simulink library "Lib_Piccolo"  (R2018b)
settings: Solver=VariableStepAuto  StartTime=0.0  StopTime=10.0  RelTol=1e-3
values from neighbouring files (symbols this model uses):
  AccelErrInt2Brakes = 0.15    [SimulationControlConfig16P.m]    (also in SimulationControlConfig16P_F0.m; SimulationControlConfig16P_F2.m; SimulationControlConfig16P_LEGACY.m; SimulationControlConfigTAILLESS.m = 0.2)
  AileronMax = 25    [SimulationControlConfig16P.m]    (also in SimulationControlConfig16P_F0.m; SimulationControlConfig16P_F2.m; SimulationControlConfig16P_LEGACY.m; SimulationControlConfigTAILLESS.m)
  AileronPower = 0.00268    [SimulationControlConfig16P.m]    (also in SimulationControlConfig16P_F0.m; SimulationControlConfig16P_F2.m; SimulationControlConfig16P_LEGACY.m; SimulationControlConfigTAILLESS.m = 0.002266)
  AileronSurfaceMax = 45    [SimulationControlConfig16P.m]    (also in SimulationControlConfig16P_F0.m; SimulationControlConfig16P_F2.m; SimulationControlConfig16P_LEGACY.m; SimulationControlConfigTAILLESS_CGAFT_F0.m = 25)
  AileronTrim = 0    [SimulationControlConfig16P.m]    (also in SimulationControlConfig16P_F0.m; SimulationControlConfig16P_F2.m; SimulationControlConfig16P_LEGACY.m; SimulationControlConfigTAILLESS.m)
  Alt = 1000 + TerrainHeight    [SimulationStateConfig.m]
  AltCruise_m = Alt * 0.3048    [SimulationControlConfig16P.m]    (also in SimulationControlConfig16P_F2.m; SimulationControlConfigTAILLESS.m = Alt/3.28084; SimulationControlConfigTAILLESS_CGAFT_F0.m = 640; SimulationControlConfigTAILLESS_CGFWD_F0.m = 640)
  AltitudeRate2PitchCmdIntegratorInit = 0.1    [SimulationControlPre.m]
  AltMax = 10000    [SimulationControlConfig16P.m]    (also in SimulationControlConfig16P_F0.m; SimulationControlConfig16P_F2.m; SimulationControlConfig16P_LEGACY.m; SimulationControlConfigTAILLESS.m)
  AltMaxAccel = 2.5    [SimulationControlConfig16P.m]    (also in SimulationControlConfig16P_F0.m = 2; SimulationControlConfig16P_F2.m = 2; SimulationControlConfig16P_LEGACY.m = 0.9; SimulationControlConfigTAILLESS.m = 2)
  AltMin = 0    [SimulationControlConfig16P.m]    (also in SimulationControlConfig16P_F0.m; SimulationControlConfig16P_F2.m; SimulationControlConfig16P_LEGACY.m; SimulationControlConfigTAILLESS.m)
  AltRateCmd2Pitch = 0.26    [SimulationControlConfig16P.m]    (also in SimulationControlConfig16P_F0.m = 0.35; SimulationControlConfig16P_F2.m = 0.35; SimulationControlConfig16P_LEGACY.m = 0.6; SimulationControlConfigTAILLESS.m = 0.9)
  AltRateError2Pitch = 0.34    [SimulationControlConfig16P.m]    (also in SimulationControlConfig16P_F0.m = 0.61; SimulationControlConfig16P_F2.m = 0.61; SimulationControlConfig16P_LEGACY.m = 0.4; SimulationControlConfigTAILLESS.m = 0.3)
  AltRateErrorInt2Pitch = 0.61    [SimulationControlConfig16P.m]    (also in SimulationControlConfig16P_F0.m = 0.28; SimulationControlConfig16P_F2.m = 0.28; SimulationControlConfig16P_LEGACY.m = 0.45; SimulationControlConfigTAILLESS.m = 0.15)
  AltRateLpfCutOff = 3    [SimulationControlConfig16P.m]    (also in SimulationControlConfig16P_F0.m; SimulationControlConfig16P_F2.m; SimulationControlConfig16P_LEGACY.m; SimulationControlConfigTAILLESS.m = 5)
  AutoNosegear2Rudder = 26    [SimulationControlConfig16P.m]    (also in SimulationControlConfig16P_F0.m; SimulationControlConfig16P_F2.m; SimulationControlConfig16P_LEGACY.m; SimulationControlConfigTAILLESS.m = 25.2)
  b = 5.54    [SimulationControlConfig16P.m]    (also in SimulationControlConfig16P_F0.m; SimulationControlConfig16P_F2.m; SimulationControlConfig16P_LEGACY.m; SimulationControlConfigTAILLESS.m = 2.37)
  Bank2AileronIntegratorInit = 0    [SimulationControlPre.m]
  BankMax_User = BankMax_User/180*pi    (= 0.610865238198)    [SimulationControlConfig16P.m]    (also in SimulationControlConfig16P_F0.m = 0.523598775598; SimulationControlConfig16P_F2.m = 0.523598775598; SimulationControlConfig16P_LEGACY.m = 0.523598775598; SimulationControlConfigTAILLESS.m = 0.558505360638)
  baseLegFlaps = 20    [SimulationControlConfig16P.m]    (also in SimulationControlConfig16P_F0.m; SimulationControlConfig16P_F2.m = 15; SimulationControlConfig16P_LEGACY.m = 0; SimulationControlConfigTAILLESS.m = 0)
  C = GeneticOpt.C    [SimulationCostFunction.m]
  c = Sw/b    (= 0.841696750903)    [SimulationControlConfig16P.m]    (also in SimulationControlConfig16P_F0.m; SimulationControlConfig16P_F2.m; SimulationControlConfig16P_LEGACY.m; SimulationControlConfigTAILLESS.m = 0.354008438819)
  cell2WheelFactorMG = 5.98    [SimulationSensorConfig16P_LEGACY.m]
  cell2WheelFactorNG = 1    [SimulationSensorConfig16P_LEGACY.m]
  cellSatMaxMG = 15000    [SimulationSensorConfig16P.m]    (also in SimulationSensorConfig16P_LEGACY.m; SimulationSensorConfigTAILLESS7P.m; SimulationSensorConfigUTAIL7P.m)
  cellSatMaxNG = 1000    [SimulationSensorConfig16P.m]    (also in SimulationSensorConfig16P_LEGACY.m; SimulationSensorConfigTAILLESS7P.m; SimulationSensorConfigUTAIL7P.m)
  cellSatMinMG = -15000    [SimulationSensorConfig16P.m]    (also in SimulationSensorConfig16P_LEGACY.m; SimulationSensorConfigTAILLESS7P.m; SimulationSensorConfigUTAIL7P.m)
  cellSatMinNG = -1000    [SimulationSensorConfig16P.m]    (also in SimulationSensorConfig16P_LEGACY.m; SimulationSensorConfigTAILLESS7P.m; SimulationSensorConfigUTAIL7P.m)
  CL_Limit = CL_Max    (= 0.54)    [SimulationControlConfig16P.m]    (also in SimulationControlConfig16P_F0.m; SimulationControlConfig16P_F2.m = 0.638; SimulationControlConfig16P_LEGACY.m; SimulationControlConfigTAILLESS.m = 0.525)
  CL_Max = 0.54    [SimulationControlConfig16P.m]    (also in SimulationControlConfig16P_F0.m; SimulationControlConfig16P_F2.m = 0.638; SimulationControlConfig16P_LEGACY.m; SimulationControlConfigTAILLESS.m = 0.525)
  CL_Max_Nom = 0.465    [SimulationControlConfig16P.m]    (also in SimulationControlConfig16P_F0.m; SimulationControlConfig16P_F2.m = 0.563; SimulationControlConfig16P_LEGACY.m; SimulationControlConfigTAILLESS.m = 0.39)
  CL_Min = 0    [SimulationControlConfig16P.m]    (also in SimulationControlConfig16P_F0.m; SimulationControlConfig16P_F2.m; SimulationControlConfig16P_LEGACY.m; SimulationControlConfigTAILLESS.m)
  ClimbMaxFraction = 0.35    [SimulationControlConfig16P.m]    (also in SimulationControlConfig16P_F0.m = 0.17; SimulationControlConfig16P_F2.m = 0.17; SimulationControlConfig16P_LEGACY.m = 0.24; SimulationControlConfigTAILLESS.m = 0.21)
  ClimboutMaxBank = 7.0    (= 7)    [SimulationControlConfig16P.m]    (also in SimulationControlConfig16P_F0.m; SimulationControlConfig16P_F2.m; SimulationControlConfig16P_LEGACY.m; SimulationControlConfigTAILLESS.m = 5)
  ClimboutTimer = 7.0    (= 7)    [SimulationControlConfig16P.m]    (also in SimulationControlConfig16P_F0.m; SimulationControlConfig16P_F2.m; SimulationControlConfig16P_LEGACY.m; SimulationControlConfigTAILLESS.m)
  dCl_per_dFlap = 0.005581818    [SimulationControlConfig16P.m]    (also in SimulationControlConfig16P_F0.m = 0; SimulationControlConfig16P_F2.m = 0.0065; SimulationControlConfig16P_LEGACY.m = 0; SimulationControlConfigTAILLESS.m = 0)
  DecelerationCmd = 3.1    [SimulationControlConfig16P.m]    (also in SimulationControlConfig16P_F0.m; SimulationControlConfig16P_F2.m; SimulationControlConfig16P_LEGACY.m; SimulationControlConfigTAILLESS.m = 0.1)
  DeRotateLogicEndTimer = abs((NoseDownLimit_Deg-1)/DeRotateRamp_Dps)    [SimulationControlConfig16P.m]    (also in SimulationControlConfig16P_F0.m; SimulationControlConfig16P_F2.m; SimulationControlConfig16P_LEGACY.m; SimulationControlConfigTAILLESS.m)
  DeRotateLogicHoldNoseUpTimer = 0.1    [SimulationControlConfig16P.m]    (also in SimulationControlConfig16P_F0.m; SimulationControlConfig16P_F2.m; SimulationControlConfig16P_LEGACY.m; SimulationControlConfigTAILLESS.m)
  DeRotateLogicTimerTimeout = 2    [SimulationControlConfig16P.m]    (also in SimulationControlConfig16P_F0.m; SimulationControlConfig16P_F2.m; SimulationControlConfig16P_LEGACY.m; SimulationControlConfigTAILLESS.m)
  DeRotateLowerCmdSaturation = 0    [SimulationControlConfig16P.m]    (also in SimulationControlConfig16P_F0.m; SimulationControlConfig16P_F2.m; SimulationControlConfig16P_LEGACY.m; SimulationControlConfigTAILLESS.m)
  DeRotateRamp_Dps = 3    [SimulationControlConfig16P.m]    (also in SimulationControlConfig16P_F0.m; SimulationControlConfig16P_F2.m; SimulationControlConfig16P_LEGACY.m; SimulationControlConfigTAILLESS.m = 8)
  DeRotateUpperCmdSaturation = 7    [SimulationControlConfig16P.m]    (also in SimulationControlConfig16P_F0.m; SimulationControlConfig16P_F2.m; SimulationControlConfig16P_LEGACY.m; SimulationControlConfigTAILLESS.m)
  DescentMaxFraction = 0.22    [SimulationControlConfig16P.m]    (also in SimulationControlConfig16P_F0.m = 0.2; SimulationControlConfig16P_F2.m = 0.2; SimulationControlConfig16P_LEGACY.m = 0.2; SimulationControlConfigTAILLESS.m = 0.17)
  DesktopSimTerrainOffset_m = 0.406    [SimulationAircraftConfig.m]
  downwindFlaps = 0    [SimulationControlConfig16P.m]    (also in SimulationControlConfig16P_F0.m; SimulationControlConfig16P_F2.m = 15; SimulationControlConfig16P_LEGACY.m; SimulationControlConfigTAILLESS.m)
  downwindSplitAil = 0    [SimulationControlConfig16P_F2.m]
  DP_init = 0.5*1.225*V_init^2    [SimulationControlConfig16P.m]    (also in SimulationControlConfig16P_F0.m; SimulationControlConfig16P_F2.m; SimulationControlConfig16P_LEGACY.m; SimulationControlConfigTAILLESS.m)
  dscNoiseMG = 1    [SimulationSensorConfig16P_LEGACY.m]
  dscNoiseNG = 0.25    [SimulationSensorConfig16P_LEGACY.m]
  DSCnumBits = 24    [SimulationSensorConfig16P.m]    (also in SimulationSensorConfig16P_LEGACY.m; SimulationSensorConfigTAILLESS7P.m; SimulationSensorConfigUTAIL7P.m)
  DSCRangeMaxMG = 15000    [SimulationSensorConfig16P.m]    (also in SimulationSensorConfig16P_LEGACY.m; SimulationSensorConfigTAILLESS7P.m; SimulationSensorConfigUTAIL7P.m)
  DSCRangeMaxNG = 1000    [SimulationSensorConfig16P.m]    (also in SimulationSensorConfig16P_LEGACY.m; SimulationSensorConfigTAILLESS7P.m; SimulationSensorConfigUTAIL7P.m)
  DSCRangeMinMG = -15000    [SimulationSensorConfig16P.m]    (also in SimulationSensorConfig16P_LEGACY.m; SimulationSensorConfigTAILLESS7P.m; SimulationSensorConfigUTAIL7P.m)
  DSCRangeMinNG = -1000    [SimulationSensorConfig16P.m]    (also in SimulationSensorConfig16P_LEGACY.m; SimulationSensorConfigTAILLESS7P.m; SimulationSensorConfigUTAIL7P.m)
  dt = DLLSim.dt    [SimulationTimeStep.m]    (also in SimulationTrim.m = 0.02)
  EarlyTouchdownThreshold = 3.0    (= 3)    [SimulationControlConfig16P.m]    (also in SimulationControlConfig16P_F0.m; SimulationControlConfig16P_F2.m; SimulationControlConfig16P_LEGACY.m; SimulationControlConfigTAILLESS.m)
  ElevatorDeflectionRate = 15    [SimulationControlConfig16P.m]    (also in SimulationControlConfig16P_F0.m; SimulationControlConfig16P_F2.m; SimulationControlConfig16P_LEGACY.m = 12; SimulationControlConfigTAILLESS.m = 5)
  ElevatorMax = 25    [SimulationControlConfig16P.m]    (also in SimulationControlConfig16P_F0.m; SimulationControlConfig16P_F2.m; SimulationControlConfig16P_LEGACY.m; SimulationControlConfigTAILLESS.m)
  ElevatorPower = -0.002209    [SimulationControlConfig16P.m]    (also in SimulationControlConfig16P_F0.m; SimulationControlConfig16P_F2.m; SimulationControlConfig16P_LEGACY.m; SimulationControlConfigTAILLESS.m = -0.002668)
  ElevatorTrim = -3.5    [SimulationControlConfig16P.m]    (also in SimulationControlConfig16P_F0.m; SimulationControlConfig16P_F2.m; SimulationControlConfig16P_LEGACY.m; SimulationControlConfigTAILLESS.m = -3)
  elevonBias = 0    [SimulationControlConfig16P.m]    (also in SimulationControlConfig16P_F0.m; SimulationControlConfig16P_F2.m; SimulationControlConfig16P_LEGACY.m; SimulationControlConfigTAILLESS.m)
  Enable_TAS_Protection = 0    [SimulationControlConfig16P.m]    (also in SimulationControlConfig16P_F0.m; SimulationControlConfig16P_F2.m; SimulationControlConfig16P_LEGACY.m; SimulationControlConfigTAILLESS.m)
  EnableCrossTrackAbort = 1    [SimulationControlConfig16P.m]    (also in SimulationControlConfigTAILLESS.m; SimulationControlConfigTAILLESS_CGAFT_F0.m; SimulationControlConfigTAILLESS_CGFWD_F0.m; SimulationControlConfigTAILLESS_CGFWD_F2.m)
  EnergyBandwidth = 0.04    [SimulationControlConfig16P.m]    (also in SimulationControlConfig16P_F0.m = 0.03; SimulationControlConfig16P_F2.m = 0.03; SimulationControlConfig16P_LEGACY.m = 0.02; SimulationControlConfigTAILLESS.m = 0.06)
  EngineLhFuelCut = 0    [SimulationAircraftConfig.m]
  EngineRhFuelCut = 0    [SimulationAircraftConfig.m]
  FastThrottleRate = 0.075    [SimulationControlConfig16P.m]    (also in SimulationControlConfig16P_F0.m = 0.05; SimulationControlConfig16P_F2.m = 0.05; SimulationControlConfig16P_LEGACY.m = 0.05; SimulationControlConfigTAILLESS.m = 0.1)
  FilterWarmUpTime = 2    [SimulationSensorConfig16P.m]    (also in SimulationSensorConfig16P_LEGACY.m; SimulationSensorConfigTAILLESS7P.m; SimulationSensorConfigUTAIL7P.m)
  finalApproachFlaps = 20    [SimulationControlConfig16P.m]    (also in SimulationControlConfig16P_F0.m; SimulationControlConfig16P_F2.m = 15; SimulationControlConfig16P_LEGACY.m = 0; SimulationControlConfigTAILLESS.m = 0)
  finalApproachSplitAil = 20    [SimulationControlConfig16P_F2.m]
  FinalDescentSlope_Deg = testPlans(testIndx).descentSlope    [SimulationControlConfig16P.m]    (also in SimulationControlConfig16P_F0.m; SimulationControlConfig16P_F2.m; SimulationControlConfig16P_LEGACY.m; SimulationControlConfigTAILLESS.m)
  flapMax = 0    [SimulationControlConfig16P.m]    (also in SimulationControlConfig16P_F0.m = 35; SimulationControlConfig16P_F2.m = 33; SimulationControlConfig16P_LEGACY.m; SimulationControlConfigTAILLESS.m)
  flapRate = 7.5    [SimulationControlConfig16P.m]    (also in SimulationControlConfig16P_F0.m; SimulationControlConfig16P_F2.m; SimulationControlConfig16P_LEGACY.m; SimulationControlConfigTAILLESS.m = 6.6)
  FlareHeight = 5    [SimulationControlConfig16P.m]    (also in SimulationControlConfig16P_F0.m; SimulationControlConfig16P_F2.m; SimulationControlConfig16P_LEGACY.m = 4.8; SimulationControlConfigTAILLESS.m = 2.75)
  FlareVerticalRate_mps = -0.4    [SimulationControlConfig16P.m]    (also in SimulationControlConfig16P_F0.m; SimulationControlConfig16P_F2.m; SimulationControlConfig16P_LEGACY.m = -0.5; SimulationControlConfigTAILLESS.m = -0.15)
  Fp_Aileron = 0.55*2*pi*RollRateLpfCutoff*dt    [SimulationControlConfig16P.m]    (also in SimulationControlConfig16P_F0.m; SimulationControlConfig16P_F2.m; SimulationControlConfig16P_LEGACY.m; SimulationControlConfigTAILLESS.m)
  Fp_Alt = 2*pi*0.55*AltBandwidth    (= 0.622035345411)    [SimulationControlConfig16P.m]    (also in SimulationControlConfig16P_F0.m; SimulationControlConfig16P_F2.m; SimulationControlConfig16P_LEGACY.m = 0.099; SimulationControlConfigTAILLESS.m = 0.207345115137)
  Fp_AltRate = 0.55*2*pi*AltRateLpfCutOff*dt    [SimulationControlConfig16P.m]    (also in SimulationControlConfig16P_F0.m; SimulationControlConfig16P_F2.m; SimulationControlConfig16P_LEGACY.m; SimulationControlConfigTAILLESS.m)
  Fp_Elevator = 0.55*2*pi*PitchRateLpfCutoff*dt    [SimulationControlConfig16P.m]    (also in SimulationControlConfig16P_F0.m; SimulationControlConfig16P_F2.m; SimulationControlConfig16P_LEGACY.m; SimulationControlConfigTAILLESS.m)
  Fp_Energy = 0.55*2*pi*EnergyBandwidth    (= 0.138230076758)    [SimulationControlConfig16P.m]    (also in SimulationControlConfig16P_F0.m = 0.103672557568; SimulationControlConfig16P_F2.m = 0.103672557568; SimulationControlConfig16P_LEGACY.m = 0.069115038379; SimulationControlConfigTAILLESS.m = 0.207345115137)
  Fp_Energy2 = 0.55*2*pi*EnergyBandwidth*dt    [SimulationControlConfig16P.m]    (also in SimulationControlConfig16P_F0.m; SimulationControlConfig16P_F2.m; SimulationControlConfig16P_LEGACY.m; SimulationControlConfigTAILLESS.m)
  Fp_Pitch = 0.55*2*pi*PitchBandwidth    (= 2.45358386245)    [SimulationControlConfig16P.m]    (also in SimulationControlConfig16P_F0.m; SimulationControlConfig16P_F2.m = 1.72787595947; SimulationControlConfig16P_LEGACY.m = 3.11017672705; SimulationControlConfigTAILLESS.m = 1.55508836353)
  Fp_Pitch_2 = 0.55*2*pi*PitchBandwidth*dt    [SimulationControlConfig16P.m]    (also in SimulationControlConfig16P_F0.m; SimulationControlConfig16P_F2.m; SimulationControlConfig16P_LEGACY.m; SimulationControlConfigTAILLESS.m)
  Fp_Roll = RollBandwidth^2    (= 1.69)    [SimulationControlConfig16P.m]    (also in SimulationControlConfig16P_F0.m = 1.44; SimulationControlConfig16P_F2.m = 1.44; SimulationControlConfig16P_LEGACY.m = 1.44; SimulationControlConfigTAILLESS.m = 1.21)
  Fp_Rudder = 0.55*2*pi*YawRateLpfCutoff*dt    [SimulationControlConfig16P.m]    (also in SimulationControlConfig16P_F0.m; SimulationControlConfig16P_F2.m; SimulationControlConfig16P_LEGACY.m; SimulationControlConfigTAILLESS.m)
  Fp_TAS = 0.55*2*pi*TASBandwidth    (= 0.103672557568)    [SimulationControlConfig16P.m]    (also in SimulationControlConfig16P_F0.m; SimulationControlConfig16P_F2.m; SimulationControlConfig16P_LEGACY.m; SimulationControlConfigTAILLESS.m = 0.172787595947)
  Fp_TAS_Filter = 2*pi*TasLpfCutoff*dt    [SimulationControlConfig16P.m]    (also in SimulationControlConfig16P_F0.m; SimulationControlConfig16P_F2.m; SimulationControlConfig16P_LEGACY.m; SimulationControlConfigTAILLESS.m)
  Fp_Turn = 0.55*2*pi*TurnErrLPFcutoff    (= 0.172787595947)    [SimulationControlConfig16P.m]    (also in SimulationControlConfig16P_F0.m = 0.0345575191895; SimulationControlConfig16P_F2.m = 0.0345575191895; SimulationControlConfig16P_LEGACY.m = 0.0345575191895; SimulationControlConfigTAILLESS.m)
  Fp_TurnDerr = 0.55*2*pi*TurnDerivativeLPFcutoff    (= 0.172787595947)    [SimulationControlConfig16P.m]    (also in SimulationControlConfig16P_F0.m = 0.0345575191895; SimulationControlConfig16P_F2.m = 0.0345575191895; SimulationControlConfig16P_LEGACY.m = 0.0345575191895; SimulationControlConfigTAILLESS.m)
  FTV = 3    [SimulationAircraftConfig.m]
  ftvStaticPositionError = 1/1.18    (= 0.847457627119)    [SimulationSensorConfig16P.m]    (also in SimulationSensorConfig16P_LEGACY.m; SimulationSensorConfigTAILLESS7P.m = 1; SimulationSensorConfigUTAIL7P.m = 1)
  g = 9.81    [SimulationStateConfig.m]
  goAroundSplitAil = 0    [SimulationControlConfig16P_F2.m]
  GustSpd_Kts = testPlans(testIndx).gustSpd    [SimulationStateConfig.m]
  GustTriggerVal = testPlans(testIndx).gustTriggerVal    [SimulationStateConfig.m]
  HeadingErr2TurnRate = 0.5    [SimulationControlConfig16P.m]    (also in SimulationControlConfig16P_F0.m; SimulationControlConfig16P_F2.m; SimulationControlConfig16P_LEGACY.m; SimulationControlConfigTAILLESS.m)
  HeadingErrDer2TurnRate = 0.3    [SimulationControlConfig16P.m]    (also in SimulationControlConfig16P_F0.m; SimulationControlConfig16P_F2.m; SimulationControlConfig16P_LEGACY.m; SimulationControlConfigTAILLESS.m)
  IASbounce = IASstall*0.8    [SimulationControlPre.m]
  IAScruiseCMD = sqrt(2*m*9.81/(1.225*Sw*CL_cruise))    [SimulationControlConfig16P.m]    (also in SimulationControlConfig16P_F0.m; SimulationControlConfig16P_F2.m; SimulationControlConfig16P_LEGACY.m; SimulationControlConfigTAILLESS.m)
  IASfinalCMD = 1.12 * IASmin    [SimulationControlConfig16P.m]    (also in SimulationControlConfig16P_F0.m = 1.14 * IASmin; SimulationControlConfig16P_F2.m = 1.10 * IASmin; SimulationControlConfig16P_LEGACY.m = 1.10 * IASmin; SimulationControlConfigTAILLESS.m = 1.14 * IASmin)
  IASflareCMD = IASstall    [SimulationControlConfig16P.m]    (also in SimulationControlConfig16P_F0.m; SimulationControlConfig16P_F2.m; SimulationControlConfig16P_LEGACY.m; SimulationControlConfigTAILLESS.m)
  IASmax = 64    [SimulationControlConfig16P.m]    (also in SimulationControlConfig16P_F0.m = 46; SimulationControlConfig16P_F2.m = 52; SimulationControlConfig16P_LEGACY.m = 46; SimulationControlConfigTAILLESS.m = 38.9)
  IASmin = sqrt(2*m*9.81/(1.225*Sw*0.9*CL_Max_Nom))    [SimulationControlConfig16P.m]    (also in SimulationControlConfig16P_F0.m; SimulationControlConfig16P_F2.m; SimulationControlConfig16P_LEGACY.m; SimulationControlConfigTAILLESS.m)
  IASshortCMD = IASstall    [SimulationControlConfig16P.m]    (also in SimulationControlConfig16P_F0.m; SimulationControlConfig16P_F2.m; SimulationControlConfig16P_LEGACY.m; SimulationControlConfigTAILLESS.m)
  IASstall = sqrt(2*m*9.81/(1.225*Sw*CL_Max))    [SimulationControlConfig16P.m]    (also in SimulationControlConfig16P_F0.m; SimulationControlConfig16P_F2.m; SimulationControlConfig16P_LEGACY.m; SimulationControlConfigTAILLESS.m)
  inFlight = 1    [SimulationControlConfig16P.m]    (also in SimulationControlConfigTAILLESS.m; SimulationControlConfigTAILLESS_CGAFT_F0.m; SimulationControlConfigTAILLESS_CGFWD_F0.m; SimulationControlConfigTAILLESS_CGFWD_F2.m)
  JetCatOffset = 5    [SimulationControlConfig16P.m]    (also in SimulationControlConfig16P_F0.m; SimulationControlConfig16P_F2.m; SimulationControlConfig16P_LEGACY.m)
  LaunchRollingElevator = -1.5    [SimulationControlConfig16P.m]    (also in SimulationControlConfig16P_F0.m; SimulationControlConfig16P_F2.m = 1.25; SimulationControlConfig16P_LEGACY.m; SimulationControlConfigTAILLESS.m = 1)
  ldg_NosegearMax = 10    [SimulationControlConfig16P.m]    (also in SimulationControlConfig16P_F0.m; SimulationControlConfig16P_F2.m; SimulationControlConfig16P_LEGACY.m; SimulationControlConfigTAILLESS.m)
  ldg_TrackVyErrInt2Nosegear = 0.1250    (= 0.125)    [SimulationControlConfig16P.m]    (also in SimulationControlConfig16P_F0.m; SimulationControlConfig16P_F2.m; SimulationControlConfig16P_LEGACY.m; SimulationControlConfigTAILLESS.m = 0.00714285714286)
  ldg_TrackVyErrPro2Nosegear = 0.35    [SimulationControlConfig16P.m]    (also in SimulationControlConfig16P_F0.m; SimulationControlConfig16P_F2.m; SimulationControlConfig16P_LEGACY.m; SimulationControlConfigTAILLESS.m = 0.0546666666667)
  ldg_TrackY2Vy = 0.07    [SimulationControlConfig16P.m]    (also in SimulationControlConfig16P_F0.m; SimulationControlConfig16P_F2.m; SimulationControlConfig16P_LEGACY.m; SimulationControlConfigTAILLESS.m = 0.17)
  ldg_Vy2NosegearScalingPower = 1.075    [SimulationControlConfig16P.m]    (also in SimulationControlConfig16P_F0.m; SimulationControlConfig16P_F2.m; SimulationControlConfig16P_LEGACY.m; SimulationControlConfigTAILLESS.m = 0.6)
  ldg_Y2VyScalingPower = 0.175    [SimulationControlConfig16P.m]    (also in SimulationControlConfig16P_F0.m; SimulationControlConfig16P_F2.m; SimulationControlConfig16P_LEGACY.m; SimulationControlConfigTAILLESS.m = 0)
  ldg_YawRate2Nosegear = 0.175    [SimulationControlConfig16P.m]    (also in SimulationControlConfig16P_F0.m; SimulationControlConfig16P_F2.m; SimulationControlConfig16P_LEGACY.m; SimulationControlConfigTAILLESS.m = 0.065)
  LiftSlope = 0.064285    [SimulationControlConfig16P.m]    (also in SimulationControlConfig16P_F0.m; SimulationControlConfig16P_F2.m; SimulationControlConfig16P_LEGACY.m; SimulationControlConfigTAILLESS.m = 0.058631)
  LPFaileronInit = 0    [SimulationControlPre.m]
  LPFclestInit = 0    [SimulationControlPre.m]
  LPFenergyFFInit = 0    [SimulationControlPre.m]
  ... (+122 more)
undefined symbols (not defined in the file or in its folder): abortFlag, alphaHPF, apmDelay, BRWNOUT, CRAWOR, CRAWUR, DiscIntNeverNeededParam, DLLSim, DLLSimStep, ECOMOR, ECOMUR, Fp_Tas, GustTrigger_HeightAgl_m, IPSTAT, LCINTEG, Ldg_Persist_Time, LOWER_FLAGS, MSG_ENABLE, NoiseStd, OLDVAL, OVERRIDE_ENABLE, OVERRIDE_VALUE, REBOOT, reversionEnable, revIASMax, revIASMin, revPitchMax, revPitchMin, revPitchRateMax, revRollMax, revRollRateMax, SAMPLE, SCALON, SensorModel, sigbuilder_block, Sim_Vx, Sim_Vy, Sim_Vz, Sim_Xpos, Sim_Ypos, Sim_Zpos, SYSOR, SYSUR, TARE, TEMPOR, TEMPUR, testIndx, testPlan, testPlans, Trim_piccoloInCmd, Trim_REFSI_FD_IN_nmodeCgShifterCmd_Flag, Trim_REFSI_FD_IN_nmodeCgShifterCmd_Ft, Trim_REFSI_FD_IN_nmodeCgShifterCmdType, Trim_REFSI_FD_IN_nmodeCgShifterNRCActive, Trim_REFSI_FD_IN_nmodeFlapLhIBCmd_Deg, Trim_REFSI_FD_IN_nmodeFlapLhOBCmd_Deg, Trim_REFSI_FD_IN_nmodeFlapRhIBCmd_Deg, Trim_REFSI_FD_IN_nmodeFlapRhOBCmd_Deg, Trim_REFSI_FD_IN_nmodeSlatLhCmd_Deg ... (+11)
libraries: simulink x1237, $bdroot x179, aerolibconvert2 x63, dspswit3 x25, aerolibatmos2 x5, simulink_extras x4, dsparch4 x2, Lib_Piccolo_Alt x2, eeGeneralControl x1, dspindex x1
(part 67 of 74)

== system Lib_Piccolo/Ground Detection Systems/WoW Wrapper/Variant Subsystem/Load Cell WoW Model 24/WOW Module/Landing Configuration/Latching Logic/Primary Latch Timer ==
  Enable/!Rst : Inport
  Compare To Constant1 : simulink/Logic and Bit Operations/Compare To Constant  relop=>  const=0  OutDataTypeStr=uint8
  Compare To Constant2 : simulink/Logic and Bit Operations/Compare To Constant  relop=>=  const=period  OutDataTypeStr=boolean
  Compare To Constant3 : simulink/Logic and Bit Operations/Compare To Constant  relop===  const=0  OutDataTypeStr=boolean
  Discrete-Time Integrator : DiscreteIntegrator  ExternalReset=level  SampleTime=-1  OutDataTypeStr=double  ICPrevOutput=DiscIntNeverNeededParam  ICPrevScaledInput=DiscIntNeverNeededParam
  Expired : Outport
  wires:
  Compare To Constant1/1 -> Discrete-Time Integrator/1
  Compare To Constant2/1 -> Expired/1
  Discrete-Time Integrator/1 -> Compare To Constant2/1
  Enable/!Rst/1 -> Compare To Constant1/1, Compare To Constant3/1
  Compare To Constant3/1 -> Discrete-Time Integrator/2

== system Lib_Piccolo/Ground Detection Systems/WoW Wrapper/Variant Subsystem/Load Cell WoW Model 24/WOW Module/Landing Configuration/Timeout Logic/1-Wheel Timeout ==
  Enable/!Rst : Inport
  Compare To Constant1 : simulink/Logic and Bit Operations/Compare To Constant  relop=>  const=0  OutDataTypeStr=uint8
  Compare To Constant2 : simulink/Logic and Bit Operations/Compare To Constant  relop=>=  const=period  OutDataTypeStr=boolean
  Compare To Constant3 : simulink/Logic and Bit Operations/Compare To Constant  relop===  const=0  OutDataTypeStr=boolean
  Discrete-Time Integrator : DiscreteIntegrator  ExternalReset=level  SampleTime=-1  OutDataTypeStr=double  ICPrevOutput=DiscIntNeverNeededParam  ICPrevScaledInput=DiscIntNeverNeededParam
  Expired : Outport
  wires:
  Compare To Constant1/1 -> Discrete-Time Integrator/1
  Compare To Constant2/1 -> Expired/1
  Discrete-Time Integrator/1 -> Compare To Constant2/1
  Enable/!Rst/1 -> Compare To Constant1/1, Compare To Constant3/1
  Compare To Constant3/1 -> Discrete-Time Integrator/2

== system Lib_Piccolo/Ground Detection Systems/WoW Wrapper/Variant Subsystem/Load Cell WoW Model 24/WOW Module/Subsystem/Comms Timeout Logic/FLAG Timeout Counter ==
  Trigger/!Rst : Inport  OutDataTypeStr=boolean
  x0 : Inport  Port=2
  Compare To Constant : simulink/Logic and Bit Operations/Compare To Constant  relop=>=  const=SensorModel.WOW.Cell.FLAG_TIMEOUT_COUNTS  OutDataTypeStr=boolean
  Custom Counter : Subsystem
  Limit Count : $bdroot/Ground Detection Systems/WoW Wrapper/Variant Subsystem/Load Cell WoW Model 20/WOW Module/Subsystem/Comms Timeout Logic/LOAD Timeout Counter/Limit Count  SystemSampleTime=-1
  NOT : Logic  Operator=NOT  IconShape=distinctive  AllPortsSameDT=off  OutDataTypeStr=boolean
  TIMEOUT : Outport
  wires:
  Custom Counter/1(Cnt) -> Compare To Constant/1  "Cnt"
  Trigger/!Rst/1 -> Limit Count/2, NOT/1
  Compare To Constant/1 -> Limit Count/1, TIMEOUT/1
  x0/1 -> Custom Counter/3(Init)
  Limit Count/1 -> Custom Counter/1(Inc)
  NOT/1 -> Custom Counter/2(Rst)

== system Lib_Piccolo/Ground Detection Systems/WoW Wrapper/Variant Subsystem/Load Cell WoW Model 24/WOW Module/Subsystem/Comms Timeout Logic/LOAD Timeout Counter ==
  Trigger/!Rst : Inport  OutDataTypeStr=boolean
  x0 : Inport  Port=2
  Compare To Constant : simulink/Logic and Bit Operations/Compare To Constant  relop=>=  const=SensorModel.WOW.Cell.LOAD_TIMEOUT_COUNTS  OutDataTypeStr=boolean
  Custom Counter : Subsystem
  Limit Count : Subsystem
  NOT : Logic  Operator=NOT  IconShape=distinctive  AllPortsSameDT=off  OutDataTypeStr=boolean
  TIMEOUT : Outport
  wires:
  NOT/1 -> Custom Counter/2(Rst)
  Limit Count/1(Inc) -> Custom Counter/1(Inc)
  x0/1 -> Custom Counter/3(Init)
  Compare To Constant/1 -> Limit Count/1(Timeout), TIMEOUT/1
  Custom Counter/1(Cnt) -> Compare To Constant/1  "Cnt"
  Trigger/!Rst/1 -> Limit Count/2(Trigger), NOT/1

== system Lib_Piccolo/Ground Detection Systems/WoW Wrapper/Variant Subsystem/Load Cell WoW Model 24/WOW Module/Subsystem/Comms Timeout Logic/Latch ==
  D : Inport
  Enable/!Rst : Inport  Port=2
  AND : Logic  IconShape=distinctive  AllPortsSameDT=off  OutDataTypeStr=boolean
  Constant : Constant  OutDataTypeStr=boolean
  OR : Logic  Operator=OR  IconShape=distinctive  AllPortsSameDT=off  OutDataTypeStr=boolean
  Switch : Switch  Criteria=u2 > Threshold  Threshold=0.5
  Unit Delay : UnitDelay  SampleTime=-1
  Q_Latched : Outport
  wires:
  Constant/1 -> Switch/1
  Enable/!Rst/1 -> AND/2
  AND/1 -> Switch/2
  OR/1 -> AND/1
  D/1 -> OR/1, Switch/3
  Switch/1 -> Unit Delay/1, Q_Latched/1
  Unit Delay/1 -> OR/2

== system Lib_Piccolo/Ground Detection Systems/WoW Wrapper/Variant Subsystem/Load Cell WoW Model 24/WOW Module/Subsystem/Comms Timeout Logic/Reset Value Selector ==
  Init : Inport  OutDataTypeStr=boolean
  Constant : Constant  Value=SensorModel.WOW.Cell.LOAD_TIMEOUT_COUNTS  OutDataTypeStr=uint8
  Constant1 : Constant  Value=SensorModel.WOW.Cell.FLAG_TIMEOUT_COUNTS  OutDataTypeStr=uint8
  Constant2 : Constant  Value=0  OutDataTypeStr=uint8
  Constant3 : Constant  Value=0  OutDataTypeStr=uint8
  Switch : Switch  Criteria=u2 > Threshold  Threshold=0.5
  Switch1 : Switch  Criteria=u2 > Threshold  Threshold=0.5
  Reset Value LOAD : Outport  OutDataTypeStr=uint8
  Reset Value FLAG : Outport  Port=2  OutDataTypeStr=uint8
  wires:
  Init/1 -> Switch1/2, Switch/2
  Constant/1 -> Switch/1
  Constant1/1 -> Switch1/1
  Switch/1 -> Reset Value LOAD/1
  Switch1/1 -> Reset Value FLAG/1
  Constant2/1 -> Switch1/3
  Constant3/1 -> Switch/3

== system Lib_Piccolo/Ground Detection Systems/WoW Wrapper/Variant Subsystem/Load Cell WoW Model 24/WOW Module/Subsystem/Health Check/DSC FLAG Decode ==
  MGR FLAG Word : Inport  OutDataTypeStr=uint16
  MGL FLAG Word : Inport  Port=2  OutDataTypeStr=uint16
  NG FLAG Word : Inport  Port=3  OutDataTypeStr=uint16
  Bus Creator : BusCreator  Inputs=TEMPUR,TEMPOR,ECOMUR,ECOMOR,CRAWUR,CRAWOR,SYSUR,SYSOR,LCINTEG,WDRST,BRWNOUT,REBOOT,LOWER_FLAGS  OutDataTypeStr=Bus: FLAG_SIGNAL_BUS  NonVirtualBus=on
  Bus Creator1 : BusCreator  Inputs=TEMPUR,TEMPOR,ECOMUR,ECOMOR,CRAWUR,CRAWOR,SYSUR,SYSOR,LCINTEG,WDRST,BRWNOUT,REBOOT,LOWER_FLAGS  OutDataTypeStr=Bus: FLAG_SIGNAL_BUS  NonVirtualBus=on
  Bus Creator2 : BusCreator  Inputs=TEMPUR,TEMPOR,ECOMUR,ECOMOR,CRAWUR,CRAWOR,SYSUR,SYSOR,LCINTEG,WDRST,BRWNOUT,REBOOT,LOWER_FLAGS  OutDataTypeStr=Bus: FLAG_SIGNAL_BUS  NonVirtualBus=on
  Extract Flags MGL : $bdroot/Ground Detection Systems/WoW Wrapper/Variant Subsystem/Load Cell WoW Model 20/WOW Module/Subsystem/Health Check/DSC FLAG Decode/Extract Flags MGR  SystemSampleTime=-1
  Extract Flags MGR : Subsystem
  Extract Flags NG : $bdroot/Ground Detection Systems/WoW Wrapper/Variant Subsystem/Load Cell WoW Model 20/WOW Module/Subsystem/Health Check/DSC FLAG Decode/Extract Flags MGR  SystemSampleTime=-1
  OR : Logic  Operator=OR  Inputs=3  IconShape=distinctive  AllPortsSameDT=off  OutDataTypeStr=boolean
  OR1 : Logic  Operator=OR  Inputs=3  IconShape=distinctive  AllPortsSameDT=off  OutDataTypeStr=boolean
  OR2 : Logic  Operator=OR  Inputs=3  IconShape=distinctive  AllPortsSameDT=off  OutDataTypeStr=boolean
  Persistence Counter : Subsystem
  Persistence Counter1 : $bdroot/Ground Detection Systems/WoW Wrapper/Variant Subsystem/Load Cell WoW Model 20/WOW Module/Subsystem/Health Check/DSC FLAG Decode/Persistence Counter  SystemSampleTime=-1
  Persistence Counter2 : $bdroot/Ground Detection Systems/WoW Wrapper/Variant Subsystem/Load Cell WoW Model 20/WOW Module/Subsystem/Health Check/DSC FLAG Decode/Persistence Counter  SystemSampleTime=-1
  MGR_FLAG_RESET : Outport
  MGL_FLAG_RESET : Outport  Port=2
  NG_FLAG_RESET : Outport  Port=3
  MGR_FLAGS : Outport  Port=4
  MGL_FLAGS : Outport  Port=5
  NG_FLAGS : Outport  Port=6
  wires:
  MGL FLAG Word/1 -> Extract Flags MGL/1
  NG FLAG Word/1 -> Extract Flags NG/1
  Extract Flags MGR/4(ECOMOR) -> Bus Creator/4, OR/2  "ECOMOR"
  Extract Flags MGR/13(LOWER_FLAGS) -> Bus Creator/13  "LOWER_FLAGS"
  Bus Creator/1 -> MGR_FLAGS/1
  Extract Flags MGR/11(BRWNOUT) -> Bus Creator/11  "BRWNOUT"
  Extract Flags MGR/10(WDRST) -> Bus Creator/10  "WDRST"
  Extract Flags MGR/8(SYSOR) -> Bus Creator/8  "SYSOR"
  Extract Flags MGR/12(REBOOT) -> Bus Creator/12  "REBOOT"
  Extract Flags MGR/1(TEMPUR) -> Bus Creator/1  "TEMPUR"
  Extract Flags MGR/9(LCINTEG) -> Bus Creator/9, OR/3  "LCINTEG"
  OR/1 -> Persistence Counter/1(Trigger/!Rst)
  Extract Flags MGR/2(TEMPOR) -> Bus Creator/2  "TEMPOR"
  Extract Flags MGR/6(CRAWOR) -> Bus Creator/6  "CRAWOR"
  Extract Flags MGR/5(CRAWUR) -> Bus Creator/5  "CRAWUR"
  Extract Flags MGR/7(SYSUR) -> Bus Creator/7  "SYSUR"
  Extract Flags MGR/3(ECOMUR) -> Bus Creator/3, OR/1  "ECOMUR"
  MGR FLAG Word/1 -> Extract Flags MGR/1(Flag Word)
  Extract Flags MGL/1 -> Bus Creator1/1  "TEMPUR"
  Extract Flags MGL/12 -> Bus Creator1/12  "REBOOT"
  Extract Flags MGL/8 -> Bus Creator1/8  "SYSOR"
  Extract Flags MGL/10 -> Bus Creator1/10  "WDRST"
  Extract Flags MGL/5 -> Bus Creator1/5  "CRAWUR"
  Extract Flags MGL/2 -> Bus Creator1/2  "TEMPOR"
  OR1/1 -> Persistence Counter1/1
  Extract Flags MGL/9 -> Bus Creator1/9, OR1/3  "LCINTEG"
  Bus Creator1/1 -> MGL_FLAGS/1
  Extract Flags MGL/6 -> Bus Creator1/6  "CRAWOR"
  Extract Flags MGL/7 -> Bus Creator1/7  "SYSUR"
  Extract Flags MGL/13 -> Bus Creator1/13  "LOWER_FLAGS"
  Extract Flags MGL/11 -> Bus Creator1/11  "BRWNOUT"
  Extract Flags MGL/4 -> Bus Creator1/4, OR1/2  "ECOMOR"
  Extract Flags MGL/3 -> Bus Creator1/3, OR1/1  "ECOMUR"
  Extract Flags NG/1 -> Bus Creator2/1  "TEMPUR"
  Extract Flags NG/12 -> Bus Creator2/12  "REBOOT"
  Extract Flags NG/8 -> Bus Creator2/8  "SYSOR"
  Extract Flags NG/10 -> Bus Creator2/10  "WDRST"
  Extract Flags NG/5 -> Bus Creator2/5  "CRAWUR"
  Extract Flags NG/2 -> Bus Creator2/2  "TEMPOR"
  OR2/1 -> Persistence Counter2/1
  Extract Flags NG/9 -> Bus Creator2/9, OR2/3  "LCINTEG"
  Bus Creator2/1 -> NG_FLAGS/1
  Extract Flags NG/6 -> Bus Creator2/6  "CRAWOR"
  Extract Flags NG/7 -> Bus Creator2/7  "SYSUR"
  Extract Flags NG/13 -> Bus Creator2/13  "LOWER_FLAGS"
  Extract Flags NG/11 -> Bus Creator2/11  "BRWNOUT"
  Extract Flags NG/4 -> Bus Creator2/4, OR2/2  "ECOMOR"
  Extract Flags NG/3 -> Bus Creator2/3, OR2/1  "ECOMUR"
  Persistence Counter/1(TIMEOUT) -> MGR_FLAG_RESET/1
  Persistence Counter1/1 -> MGL_FLAG_RESET/1
  Persistence Counter2/1 -> NG_FLAG_RESET/1

== system Lib_Piccolo/Ground Detection Systems/WoW Wrapper/Variant Subsystem/Load Cell WoW Model 24/WOW Module/Subsystem/Health Check/DSC STAT Decode ==
  MGR STAT Word : Inport
  MGL STAT Word : Inport  Port=2
  NG STAT Word : Inport  Port=3
  Bus Creator : BusCreator  Inputs=IPSTAT,TEMPUR,TEMPOR,ECOMUR,ECOMOR,CRAWUR,CRAWOR,SYSUR,SYSOR,LCINTEG,SCALON,OLDVAL  OutDataTypeStr=Bus: STAT_SIGNAL_BUS  NonVirtualBus=on
  Bus Creator1 : BusCreator  Inputs=IPSTAT,TEMPUR,TEMPOR,ECOMUR,ECOMOR,CRAWUR,CRAWOR,SYSUR,SYSOR,LCINTEG,SCALON,OLDVAL  OutDataTypeStr=Bus: STAT_SIGNAL_BUS  NonVirtualBus=on
  Bus Creator2 : BusCreator  Inputs=IPSTAT,TEMPUR,TEMPOR,ECOMUR,ECOMOR,CRAWUR,CRAWOR,SYSUR,SYSOR,LCINTEG,SCALON,OLDVAL  OutDataTypeStr=Bus: STAT_SIGNAL_BUS  NonVirtualBus=on
  Extract STAT MGL : $bdroot/Ground Detection Systems/WoW Wrapper/Variant Subsystem/Load Cell WoW Model 20/WOW Module/Subsystem/Health Check/DSC STAT Decode/Extract STAT MGR  SystemSampleTime=-1
  Extract STAT MGR : Subsystem
  Extract STAT NG : $bdroot/Ground Detection Systems/WoW Wrapper/Variant Subsystem/Load Cell WoW Model 20/WOW Module/Subsystem/Health Check/DSC STAT Decode/Extract STAT MGR  SystemSampleTime=-1
  MGR_STAT : Outport  OutDataTypeStr=Bus: STAT_SIGNAL_BUS
  MGL_STAT : Outport  Port=2  OutDataTypeStr=Bus: STAT_SIGNAL_BUS
  NG_STAT : Outport  Port=3  OutDataTypeStr=Bus: STAT_SIGNAL_BUS
  wires:
  MGR STAT Word/1 -> Extract STAT MGR/1(STAT Word)
  MGL STAT Word/1 -> Extract STAT MGL/1
  NG STAT Word/1 -> Extract STAT NG/1
  Extract STAT MGR/1(IPSTAT) -> Bus Creator/1  "IPSTAT"
  Extract STAT MGR/2(TEMPUR) -> Bus Creator/2  "TEMPUR"
  Extract STAT MGR/3(TEMPOR) -> Bus Creator/3  "TEMPOR"
  Extract STAT MGR/4(ECOMUR) -> Bus Creator/4  "ECOMUR"
  Extract STAT MGR/5(ECOMOR) -> Bus Creator/5  "ECOMOR"
  Extract STAT MGR/6(CRAWUR) -> Bus Creator/6  "CRAWUR"
  Extract STAT MGR/7(CRAWOR) -> Bus Creator/7  "CRAWOR"
  Extract STAT MGR/8(SYSUR) -> Bus Creator/8  "SYSUR"
  Extract STAT MGR/9(SYSOR) -> Bus Creator/9  "SYSOR"
  Extract STAT MGR/10(LCINTEG) -> Bus Creator/10  "LCINTEG"
  Extract STAT MGR/11(SCALON) -> Bus Creator/11  "SCALON"
  Extract STAT MGR/12(OLDVAL) -> Bus Creator/12  "OLDVAL"
  Bus Creator/1 -> MGR_STAT/1
  Extract STAT MGL/1 -> Bus Creator1/1  "IPSTAT"
  Extract STAT MGL/2 -> Bus Creator1/2  "TEMPUR"
  Extract STAT MGL/3 -> Bus Creator1/3  "TEMPOR"
  Extract STAT MGL/4 -> Bus Creator1/4  "ECOMUR"
  Extract STAT MGL/5 -> Bus Creator1/5  "ECOMOR"
  Extract STAT MGL/6 -> Bus Creator1/6  "CRAWUR"
  Extract STAT MGL/7 -> Bus Creator1/7  "CRAWOR"
  Extract STAT MGL/8 -> Bus Creator1/8  "SYSUR"
  Extract STAT MGL/9 -> Bus Creator1/9  "SYSOR"
  Extract STAT MGL/10 -> Bus Creator1/10  "LCINTEG"
  Extract STAT MGL/11 -> Bus Creator1/11  "SCALON"
  Extract STAT MGL/12 -> Bus Creator1/12  "OLDVAL"
  Bus Creator1/1 -> MGL_STAT/1
  Extract STAT NG/1 -> Bus Creator2/1  "IPSTAT"
  Extract STAT NG/2 -> Bus Creator2/2  "TEMPUR"
  Extract STAT NG/3 -> Bus Creator2/3  "TEMPOR"
  Extract STAT NG/4 -> Bus Creator2/4  "ECOMUR"
  Extract STAT NG/5 -> Bus Creator2/5  "ECOMOR"
  Extract STAT NG/6 -> Bus Creator2/6  "CRAWUR"
  Extract STAT NG/7 -> Bus Creator2/7  "CRAWOR"
  Extract STAT NG/8 -> Bus Creator2/8  "SYSUR"
  Extract STAT NG/9 -> Bus Creator2/9  "SYSOR"
  Extract STAT NG/10 -> Bus Creator2/10  "LCINTEG"
  Extract STAT NG/11 -> Bus Creator2/11  "SCALON"
  Extract STAT NG/12 -> Bus Creator2/12  "OLDVAL"
  Bus Creator2/1 -> NG_STAT/1

== system Lib_Piccolo/Ground Detection Systems/WoW Wrapper/Variant Subsystem/Load Cell WoW Model 24/WOW Module/Subsystem/Health Check/MGR DSC Fail Logic ==
  PIC_AP_MODE : Inport
  WOW_N : Inport  Port=2
  LOAD_TIMEOUT : Inport  Port=3
  FLAG_RESET : Inport  Port=4
  FLAG_TIMEOUT : Inport  Port=5
  Bus Creator : BusCreator  Inputs=8  OutDataTypeStr=Bus: HEALTH_SIGNAL_BUS  NonVirtualBus=on
  Constant : Constant  Value=0  OutDataTypeStr=boolean
  Latch : Subsystem
  Latch Activation on Mode : $bdroot/Ground Detection Systems/WoW Wrapper/Variant Subsystem/Load Cell WoW Model 20/WOW Module/Flag Latch/Latch Activation on Mode  SystemSampleTime=-1
  MG Data Validation : Subsystem
  OR3 : Logic  Operator=OR  Inputs=5  IconShape=distinctive  AllPortsSameDT=off  OutDataTypeStr=boolean
  DSC_FAIL : Outport
  MGR_HEALTH : Outport  Port=2
  wires:
  WOW_N/1 -> MG Data Validation/2(WOW_N)
  OR3/1 -> Latch/1(D)
  FLAG_RESET/1 -> Bus Creator/6, OR3/5  "FLAG_ERROR"
  MG Data Validation/1(INVALID) -> Bus Creator/1, OR3/1  "INVALID"
  Bus Creator/1 -> MGR_HEALTH/1
  LOAD_TIMEOUT/1 -> Bus Creator/4, OR3/3  "LOAD_TIMEOUT"
  MG Data Validation/2(IN_FLIGHT_BIAS) -> Bus Creator/2  "IN_FLIGHT_BIAS"
  Latch Activation on Mode/1 -> Latch/2(Enable/!Rst)
  PIC_AP_MODE/1 -> Latch Activation on Mode/1, MG Data Validation/1(AP Mode)
  Latch/1(Q_Latched) -> Bus Creator/8, DSC_FAIL/1  "FAIL"
  FLAG_TIMEOUT/1 -> Bus Creator/5, OR3/4  "FLAG_TIMEOUT"
  MG Data Validation/3(FINAL_BIAS) -> OR3/2, Bus Creator/3  "FINAL_BIAS"
  Constant/1 -> Bus Creator/7  "ACTIVE"

== system Lib_Piccolo/Ground Detection Systems/WoW Wrapper/Variant Subsystem/Load Cell WoW Model 24/WOW Module/Subsystem/Health Check/NG DSC Fail Logic ==
  PIC_AP_MODE : Inport
  WOW_N : Inport  Port=2
  LOAD_TIMEOUT : Inport  Port=3
  FLAG_RESET : Inport  Port=4
  FLAG_TIMEOUT : Inport  Port=5
  Bus Creator : BusCreator  Inputs=8  OutDataTypeStr=Bus: HEALTH_SIGNAL_BUS  NonVirtualBus=on
  Constant : Constant  Value=0  OutDataTypeStr=boolean
  Latch : Subsystem
  Latch Activation on Mode : $bdroot/Ground Detection Systems/WoW Wrapper/Variant Subsystem/Load Cell WoW Model 20/WOW Module/Flag Latch/Latch Activation on Mode  SystemSampleTime=-1
  NG Data Validation : Subsystem
  OR3 : Logic  Operator=OR  Inputs=5  IconShape=distinctive  AllPortsSameDT=off  OutDataTypeStr=boolean
  DSC_FAIL : Outport
  MGR_HEALTH : Outport  Port=2
  wires:
  WOW_N/1 -> NG Data Validation/2(WOW_N)
  OR3/1 -> Latch/1(D)
  FLAG_RESET/1 -> Bus Creator/6, OR3/5  "FLAG_ERROR"
  NG Data Validation/1(INVALID) -> Bus Creator/1, OR3/1  "INVALID"
  Bus Creator/1 -> MGR_HEALTH/1
  LOAD_TIMEOUT/1 -> Bus Creator/4, OR3/3  "LOAD_TIMEOUT"
  NG Data Validation/2(IN_FLIGHT_BIAS) -> Bus Creator/2  "IN_FLIGHT_BIAS"
  Latch Activation on Mode/1 -> Latch/2(Enable/!Rst)
  PIC_AP_MODE/1 -> Latch Activation on Mode/1, NG Data Validation/1(AP Mode)
  Latch/1(Q_Latched) -> Bus Creator/8, DSC_FAIL/1  "FAIL"
  FLAG_TIMEOUT/1 -> Bus Creator/5, OR3/4  "FLAG_TIMEOUT"
  NG Data Validation/3(FINAL_BIAS) -> OR3/2, Bus Creator/3  "FINAL_BIAS"
  Constant/1 -> Bus Creator/7  "ACTIVE"

== system Lib_Piccolo/Ground Detection Systems/WoW Wrapper/Variant Subsystem/Load Cell WoW Model 20/WOW Module/Subsystem/Comms Timeout Logic/FLAG Timeout Counter/Custom Counter ==
  note: Custom counter with initial condition exposed as an input.
  Inc : Inport  OutDataTypeStr=boolean
  Rst : Inport  Port=2  OutDataTypeStr=boolean
  Init : Inport  Port=3  OutDataTypeStr=uint8
  Data Type Conversion : DataTypeConversion  OutDataTypeStr=uint8
  Memory : Memory  InitialCondition=SensorModel.WOW.Cell.FLAG_TIMEOUT_COUNTS
  Sum : Sum  Inputs=|++
  Switch : Switch  Criteria=u2 > Threshold  Threshold=0.5
  Cnt : Outport  OutDataTypeStr=uint8
  wires:
  Data Type Conversion/1 -> Sum/1
  Sum/1 -> Switch/3
  Rst/1 -> Switch/2
  Switch/1 -> Cnt/1, Memory/1
  Init/1 -> Switch/1
  Memory/1 -> Sum/2
  Inc/1 -> Data Type Conversion/1

== system Lib_Piccolo/Ground Detection Systems/WoW Wrapper/Variant Subsystem/Load Cell WoW Model 20/WOW Module/Subsystem/Comms Timeout Logic/LOAD Timeout Counter/Custom Counter ==
  note: Custom counter with initial condition exposed as an input.
  Inc : Inport  OutDataTypeStr=boolean
  Rst : Inport  Port=2  OutDataTypeStr=boolean
  Init : Inport  Port=3  OutDataTypeStr=uint8
  Data Type Conversion : DataTypeConversion  OutDataTypeStr=uint8
  Memory : Memory  InitialCondition=SensorModel.WOW.Cell.LOAD_TIMEOUT_COUNTS
  Sum : Sum  Inputs=|++
  Switch : Switch  Criteria=u2 > Threshold  Threshold=0.5
  Cnt : Outport  OutDataTypeStr=uint8
  wires:
  Inc/1 -> Data Type Conversion/1
  Memory/1 -> Sum/2
  Init/1 -> Switch/1
  Switch/1 -> Memory/1, Cnt/1
  Rst/1 -> Switch/2
  Sum/1 -> Switch/3
  Data Type Conversion/1 -> Sum/1

== system Lib_Piccolo/Ground Detection Systems/WoW Wrapper/Variant Subsystem/Load Cell WoW Model 20/WOW Module/Subsystem/Comms Timeout Logic/LOAD Timeout Counter/Limit Count ==
  note: If timeout condition has already been met, and trigger input is still active, dont increment the counter further.
      |
      | This prevents the counter from free-running during a sustained trigger condition, so we can use an 8-bit datatype without worrying about overflow.
  Timeout : Inport
  Trigger : Inport  Port=2
  AND : Logic  IconShape=distinctive  AllPortsSameDT=off  OutDataTypeStr=boolean
  Constant : Constant  Value=0  OutDataTypeStr=boolean
  Switch : Switch  Criteria=u2 > Threshold  Threshold=0.5
  Unit Delay : UnitDelay  SampleTime=-1
  Inc : Outport
  wires:
  Unit Delay/1 -> AND/1
  Trigger/1 -> Switch/3, AND/2
  Constant/1 -> Switch/1
  AND/1 -> Switch/2
  Timeout/1 -> Unit Delay/1
  Switch/1 -> Inc/1
